simulink model "TP3_5"  (R2018a)
settings: Solver=VariableStepAuto  StartTime=0.0  StopTime=10.0  RelTol=1e-3
libraries: dsparch4 x2
settings Model: Creator=LENOVO  LastModifiedBy=10RS5

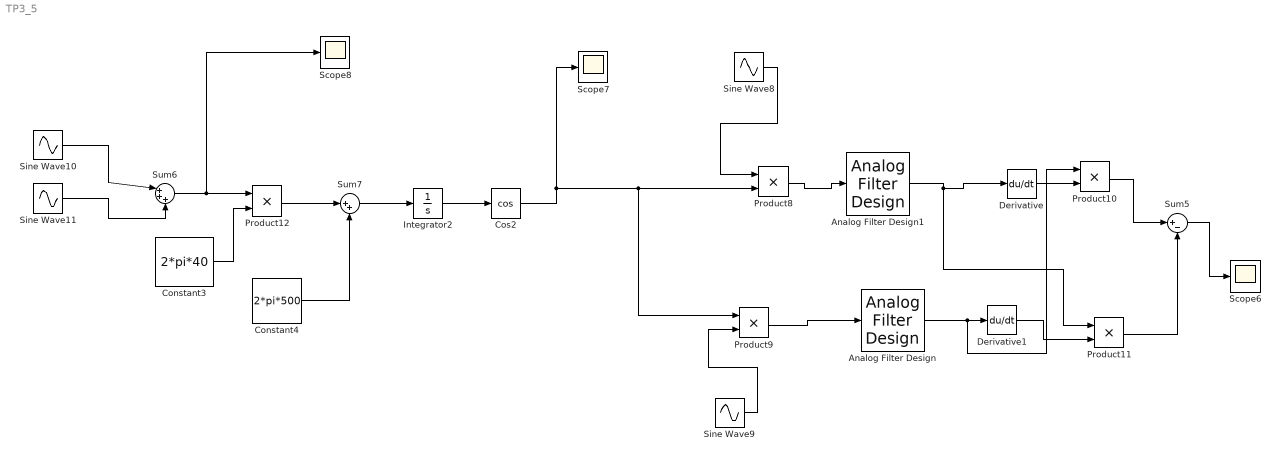
== system TP3_5 ==
  Analog Filter Design : dsparch4/Analog Filter Design  method=Butterworth  filttype=Lowpass  N=8  Wlo=500  Whi=80  Rp=2  Rs=40
  Analog Filter Design1 : dsparch4/Analog Filter Design  method=Butterworth  filttype=Lowpass  N=8  Wlo=500  Whi=80  Rp=2  Rs=40
  Constant3 : Constant  Value=2*pi*40
  Constant4 : Constant  Value=2*pi*500
  Cos2 : Trigonometry  Operator=cos
  Derivative : Derivative
  Derivative1 : Derivative
  Integrator2 : Integrator
  Product{8..12} (5 alike) : Product
  Scope6 : Scope
  Scope7 : Scope
  Scope8 : Scope
  Sine Wave10 : Sin  Frequency=10*pi  SampleTime=0
  Sine Wave11 : Sin  Amplitude=0.5  Frequency=20*pi  SampleTime=0
  Sine Wave8 : Sin  Frequency=2*pi*500  Phase=pi/2  SampleTime=0
  Sine Wave9 : Sin  Frequency=2*pi*500  SampleTime=0
  Sum5 : Sum  Inputs=|+-
  Sum6 : Sum  Inputs=|+++
  Sum7 : Sum  Inputs=|++
  wires:
  Product11/1 -> Sum5/2
  Sum6/1 -> Scope8/1, Product12/1
  Sine Wave11/1 -> Sum6/3
  Sum7/1 -> Integrator2/1
  Product10/1 -> Sum5/1
  Constant3/1 -> Product12/2
  Cos2/1 -> Scope7/1, Product9/1, Product8/2
  Constant4/1 -> Sum7/2
  Sum5/1 -> Scope6/1
  Sine Wave10/1 -> Sum6/1
  Derivative/1 -> Product10/2
  Sine Wave9/1 -> Product9/2
  Integrator2/1 -> Cos2/1
  Product8/1 -> Analog Filter Design1/1
  Derivative1/1 -> Product11/2
  Product12/1 -> Sum7/1
  Analog Filter Design1/1 -> Product11/1, Derivative/1
  Product9/1 -> Analog Filter Design/1
  Sine Wave8/1 -> Product8/1
  Analog Filter Design/1 -> Derivative1/1, Product10/1
